simulink model "sim_model_64bit"  (Simulink 9.2)
settings: Solver=ode45  StartTime=0  StopTime=18.005  RelTol=0.001  EnableMultiTasking=on
libraries: fmu_me_lib x1
settings Model: Creator=Tin Rabuzin  LastModifiedBy=meagh
settings DataIOCC: SignalLoggingSaveFormat=Dataset  OutputSaveName=simout  OutputOption=SpecifiedOutputTimes  OutputTimes=[0:0.0048:18.005]
settings OptimizationCC: ExpressionDepthLimit=2147483647
settings DebuggingCC: FcnCallInpInsideContextMsg=error
settings GRTTargetCC: CombineOutputUpdateFcns=on  GRTInterface=off

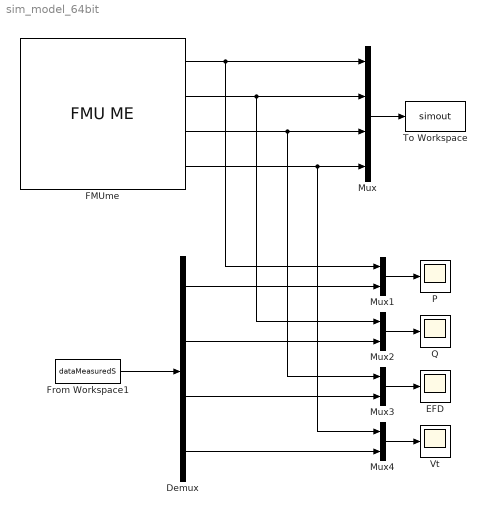
== system sim_model_64bit ==
  Demux : Demux
  EFD : Scope
  FMUme : fmu_me_lib/FMU ME  Description=Simulates an FMU for Model Exchange 1.0 or Model Exchange 2.0.  dummy=0
  From Workspace1 : FromWorkspace  VariableName=dataMeasuredS  SampleTime=0
  Mux : Mux
  Mux{1..4} (4 alike) : Mux  Inputs=2
  P : Scope
  Q : Scope
  To Workspace : ToWorkspace  VariableName=simout  SaveFormat=Structure With Time  SampleTime=-1
  Vt : Scope
  wires:
  Mux/1 -> To Workspace/1
  From Workspace1/1 -> Demux/1
  Mux1/1 -> P/1
  Mux2/1 -> Q/1
  Mux3/1 -> EFD/1
  Mux4/1 -> Vt/1
  FMUme/1 -> Mux1/1, Mux/1
  FMUme/2 -> Mux2/1, Mux/2
  FMUme/3 -> Mux3/1, Mux/3
  FMUme/4 -> Mux4/1, Mux/4
  Demux/1 -> Mux1/2
  Demux/2 -> Mux2/2
  Demux/3 -> Mux3/2
  Demux/4 -> Mux4/2
